simulink model "Scenario_MinimumExample_TwithoutTrafficLights"  (R2021a)
settings: Solver=VariableStepAuto  StartTime=0.0  StopTime=15  RelTol=1e-3
model workspace (MAT data in the model file):
  Kz_dif : Simulink.Parameter (value not decoded)
  Kz_il : Simulink.Parameter (value not decoded)
  Kz_ir : Simulink.Parameter (value not decoded)
  Kz_is : Simulink.Parameter (value not decoded)
  Kz_long : Simulink.Parameter (value not decoded)
  Kz_pre : Simulink.Parameter (value not decoded)
  L_dif : Simulink.Parameter (value not decoded)
  L_il : Simulink.Parameter (value not decoded)
  L_ir : Simulink.Parameter (value not decoded)
  L_is : Simulink.Parameter (value not decoded)
  L_long : Simulink.Parameter (value not decoded)
  L_pre : Simulink.Parameter (value not decoded)
  Lc : Simulink.Parameter (value not decoded)
  Rk : Simulink.Parameter (value not decoded)
  Tz_dif : Simulink.Parameter (value not decoded)
  Tz_il : Simulink.Parameter (value not decoded)
  Tz_ir : Simulink.Parameter (value not decoded)
  Tz_is : Simulink.Parameter (value not decoded)
  Tz_long : Simulink.Parameter (value not decoded)
  Tz_pre : Simulink.Parameter (value not decoded)
  ds : Simulink.Parameter (value not decoded)
  dt : Simulink.Parameter (value not decoded)
  v : Simulink.Parameter (value not decoded)
symbols that are objects in the model workspace (value not decoded): Kz_dif, Kz_il, Kz_ir, Kz_is, Kz_long, Kz_pre, Rk, Tz_dif, Tz_il, Tz_ir, Tz_is, Tz_long, Tz_pre
libraries: StreetLanesLibrary x72, EdgesLibrary x64, SourcesAndSinksLibrary x12
(part 2 of 3)

== stateflow chart Scenario_MinimumExample_TwithoutTrafficLights/Chart1 ==
  note: Notizen (mal auf Deutsch):
      | wenn an einer kante etwas anliegt und keine der stärkeren kanten etwas anliegen hat,
      | und die konfliktbereiche frei sind: schalte kante frei
      | <Ali 3> wird dominiert von <Cl 7> und <Cs 8> [Kreuzungen: <Brs Co> <Cl Ao> <Cs Bo>
      | <Ari 4> wird nicht dominiert [Kreuzungen: <Brs Co>
      | <Cl 7> wird dominiert von <Brs 11> und <Brs 12> [Kreuzungen: <Brs Co> <Brs Ao><Ali Bo>
      | <Cs 8> wird nicht dominiert [Kreuzungen: <Ali Bo>
      | <Brs 11> wird dominiert von <Ali 3> und <Ari 4> [Kreuzungen: <Brs Ao> <Ali Bo> <Ari Co>*<Cl Ao>
      | <Brs 12> wird nicht dominiert [Kreuzungen: <Cl Ao>
      |
      | Anmerkung: die einflüsse Brs11 und Brs12 behindern sich nicht. da beide kanten an
      | EIN UND DEMSELBEN SEGMENT liegen, und unsere 0.5:0.5 gewichtung schon suggeriert,
      | dass sich hier die autos "spalten", können sich die autos beim "Parallelen" fließen
      | in die segmente <Brs Co> und <Brs Ao> nicht wirklich in die quere kommen. Oder selbst wenn sie es
      | tun, können wir nichts dagegen unternehmen - wenn wir einem der pfade gegenüber dem anderen
      | priorität geben, wird bei dem anderen jeweils NIE etwas fließen. Damit müssen wir wohl leben :(
      |
      | a)
      | if [Ali > 0 && Cl == 0 && Cs == 0 && Brs_Co == 0 && Cl_Ao == 0 && Cs_Bo == 0]{enableAli3=1;}
      | else {enableAli3=0;}
      | b)
      | if [Ari > 0 && Brs_Co == 0]{enableAri4=1;}
      | else {enableAri4=0;}
      | c)
      | if [Cl > 0 && Brs == 0 && Brs_Co == 0 && Brs_Ao == 0 && Ali_Bo == 0]{enableCl7=1;}
      | else {enableCl7=0;}
      | d)
      | if [Cs > 0 && Ali_Bo == 0]{enableCs8=1;}
      | else {enableCs8=0;}
      | e)
      | if [Brs > 0 && Ali == 0 && Ari == 0 && Ali_Bo == 0 && Ari_Co == 0 && Cl_Ao]{enableBrs11=1;}
      | else {enableBrs11=0;}
      | f)
      | if [Brs > 0 && Cl_Ao == 0]{enableBrs12=1;}
      | else {enableBrs12=0;}
      |
      | Anmerkung: Da es im Falle [Ali > 0 && Brs > 0 && Cl > 0] einen deadlock gibt, müssen wir uns entscheiden, wer fahren darf.
      |
      | // Brs11 soll das fahrtrecht bekommen, um den fluss entlang der geraden aufrechtzuerhalten, wenn möglich
      | if [Ari == 0 && (Ali_Bo == 0 && Ari_Co == 0 && Cl_Ao == 0)]{enableBrs11=1;}
      | else
      |
      | // falls Brs12 nicht kann, versucht Ali zu fahren. Eigentlich müsste Cl die nächstbeste Wahl sein,
      | // allerdings kann Cl im falle eines Deadlocks ohnehin nicht fließen, da wegen unserer modellierung
      | // der 1x2 kanten (bzw. 1x2 segmente) gilt "Deadlock => [Brs > 0] => [Brs12 will aktiv sein]" - und da
      | // Brs12 vorrang vor Cl7 hat, ist Cl7 in diesem szenario grundsätzlich blockiert.
      | if [Cs == 0 && (Brs_Co == 0 && Cl_Ao == 0 && Cs_Bo == 0)]{enableAli3=1;}
      | else //guess noone can make it
  note: ?
  state InitiatePerStepCheck
  note: Brs-11-<Brs Co>-6-Co
      | (Links will geradeaus)
  note: Brs-12-<Brs Ao>-1-Ao
      | (Links will geradeaus)
  note: Ari-4-<Ari Co>-5-Co
      | (Unten will rechts abbiegen)
  note: Cl-7-<Cl Ao>-2-Ao
      | (Rechts will links abbiegen)
  note: Cs-8-<Cl Ao>-9-Bo
      | (Rechts will geradeaus)
  note: Ali-3-<Ali Bo>-10-Bo
      | (Unten will Links abbiegen)
  note: Deadlock-Detection
  note: Anstelle der ebene für deadlock resolution konnte man den "Links will geradeaus" bereich in der reihenfolge VOR "Unten will links abbiegen" setzen. "Links will geradeaus" muss dann um eine weitere kante mit höchster priorität ergänzt werden mit einem label
      | [ (Ali > 0 && Brs > 0 && Cl > 0 ) && (Ari == 0 && Ali_Bo == 0 && Ari_Co == 0]{enableBrs11=1;}
      |
      | "Unten will links abbiegen" wird dann ebenfalls um eine Kante mit höchster priorität ergänzt mit dem Label
      | [ (Ali > 0 && Brs > 0 && Cl > 0) && (Cs_Bo == 0 && Cl_Ao == 0) && ~(enableBrs11==1)
  note: Deadlock-Resolution
  InitiatePerStepCheck -> (junction 23) [order 1] : [Ali > 0 && Cl == 0 && Cs == 0 && Brs_Co == 0 && Cl_Ao == 0 && Cs_Bo == 0]
      | {enableAli3=1; }
  (junction 23) -> (junction 29) [order 1] : [Ari > 0 && Brs_Co == 0]{enableAri4=1;}
  (junction 29) -> (junction 36) [order 1] : [Cl > 0 && Brs == 0 && Brs_Co == 0 && Brs_Ao == 0 && Ali_Bo == 0]{enableCl7=1; }
  (junction 39) -> (junction 40) [order 1] : [Brs > 0 && Ali == 0 && Ari == 0 && Ali_Bo == 0 && Ari_Co == 0 && Cl_Ao]{enableBrs11=1;}
  (junction 40) -> (junction 45) [order 1] : [Brs > 0 && Cl_Ao == 0]{enableBrs12=1;}
  (junction 36) -> (junction 39) [order 1] : [Cs > 0 && Ali_Bo == 0]{enableCs8=1;}
  (junction 39) -> (junction 40) [order 2] : {enableBrs11=0;}
  (junction 29) -> (junction 36) [order 2] : {enableCl7=0;}
  (junction 36) -> (junction 39) [order 2] : {enableCs8=0;}
  (junction 23) -> (junction 29) [order 2] : {enableAri4=0;}
  (junction 40) -> (junction 45) [order 2] : {enableBrs12=0;}
  InitiatePerStepCheck -> (junction 23) [order 2] : {enableAli3=0;}
  (junction 45) -> (junction 53)
  (junction 53) -> InitiatePerStepCheck [order 2]
  (default) -> InitiatePerStepCheck : {enableAli3 = 0; enableAri4 = 0;
      | enableCl7 = 0; enableCs8 = 0;
      | enableBrs11 = 0; enableBrs12 = 0;}
  (junction 53) -> (junction 64) [order 1] : [Ali > 0 && Brs > 0 && Cl > 0]
  (junction 64) -> (junction 71) [order 1] : [Ari == 0 && (Ali_Bo == 0 && Ari_Co == 0 && Cl_Ao == 0)]{enableBrs11=1;}
  (junction 64) -> (junction 71) [order 2] : [Ari > 0 && Cs == 0 && (Brs_Co == 0 && Cl_Ao == 0 && Cs_Bo == 0)]{enableAli3=1;}
  (junction 71) -> InitiatePerStepCheck
  data: Ali input; Ari input; Cl input; Cs input; Brs input; Ali_Bo input; Ari_Co input; Cl_Ao input; Cs_Bo input; Brs_Co input; Brs_Ao input; enableAli3 output; enableAri4 output; enableCl7 output; enableCs8 output; enableBrs11 output; enableBrs12 output

== stateflow chart Scenario_MinimumExample_TwithoutTrafficLights/Plus-Controller ==
  note: ?
  state Group__Crs_Brs
  state Group__Cl_Bl
  state Group__Ars_Drs
  state Group__Al_Dl
  note: check
      | Crs straight
      | crossings
  note: check
      | Cl
      | crossings
  note: check
      | Ars straight
      | crossings
  note: check
      | Al
      | crossings
  note: check
      | Crs right
      | crossings
  note: check
      | Bl
      | crossings
  note: check
      | Ars right
      | crossings
  note: check
      | Dl
      | crossings
  note: check
      | Brs straight
      | crossings
  note: check
      | Drs straight
      | crossings
  note: check
      | Brs right
      | crossings
  note: check
      | Drs right
      | crossings
  Group__Al_Dl -> Group__Crs_Brs [order 2] : [[[after(green_duration_l, sec)]]]
      | {enAl = 0; enDl = 0;}
  Group__Ars_Drs -> Group__Al_Dl [order 1] : [[after(green_duration_sr, sec)]]
      | {enAs = 0; enAr = 0; enDs = 0; enDr = 0;}
  Group__Cl_Bl -> Group__Ars_Drs [order 1] : [after(green_duration_l, sec)]
      | {enCl = 0; enBl = 0;}
  Group__Crs_Brs -> Group__Cl_Bl [order 1] : [after(green_duration_sr, sec)]
      | {enCs = 0; enCr = 0; ...
      | enBs = 0; enBr = 0;}
  (default) -> Group__Crs_Brs : {enAl = 0; enAs = 0; enAr = 0;
      | enBl = 0; enBs = 0; enBr = 0;
      | enCl = 0; enCs = 0; enCr = 0;
      | enDl = 0; enDs = 0; enDr = 0;}
  Group__Crs_Brs -> (junction 51) [order 2]
  (junction 109) -> Group__Crs_Brs
  Group__Cl_Bl -> (junction 117) [order 2]
  (junction 126) -> Group__Cl_Bl
  Group__Ars_Drs -> (junction 134) [order 2]
  (junction 131) -> Group__Ars_Drs
  Group__Al_Dl -> (junction 151) [order 1]
  (junction 160) -> Group__Al_Dl
  (junction 117) -> (junction 116) [order 2] : {enCl = 0;}
  (junction 51) -> (junction 59) [order 1] : [(Dl_Co==0 && Drs_Ao==0 ...
      | && Drs_Bo==0 && Bl_Do==0 ...
      | && Al_Bo==0 && Ars_Do==0)]
      | {enCs = 1;}
  (junction 117) -> (junction 116) [order 1] : [(Dl_Co==0 && Drs_Ao==0 && ....
      | Brs_Co==0 && Al_Bo==0 && ...
      | Ars_Do==0)]{enCl = 1;}
  (junction 51) -> (junction 59) [order 2] : {enCs = 0;}
  (junction 134) -> (junction 133) [order 1] : [((Cl_Ao==0 && Crs_Bo==0 && ...
      | Crs_Do==0 && Dl_Co==0 && ...
      | Bl_Do==0 && Brs_Co==0))]
      | {enAs = 1;}
  (junction 151) -> (junction 150) [order 1] : [(Cl_Ao==0 && Crs_Bo==0 ...
      | && Drs_Ao==0 && Bl_Do==0 ...
      | && Brs_Co==0)]{enAl = 1;}
  (junction 134) -> (junction 133) [order 2] : {enAs = 0;}
  (junction 151) -> (junction 150) [order 2] : {enAl = 0;}
  (junction 59) -> (junction 104) [order 1] : [(Ars_Do==0 && Bl_Do==0)]
      | {enCr = 1;}
  (junction 116) -> (junction 126) [order 1] : [(Al_Bo==0 && Ars_Do==0 && ...
      | Crs_Bo==0 && Dl_Co==0 && ...
      | Drs_Ao==0)]{enBl = 1;}
  (junction 59) -> (junction 104) [order 2] : {enCr = 0;}
  (junction 116) -> (junction 126) [order 2] : {enBl = 0;}
  (junction 133) -> (junction 143) [order 1] : [(Brs_Co==0 && Dl_Co==0)]
      | {enAr = 1;}
  (junction 150) -> (junction 160) [order 1] : [(Bl_Do==0 && Brs_Co==0 ...
      | && Ars_Do==0 && Cl_Ao==0 ...
      | && Crs_Bo==0)]{enDl = 1;}
  (junction 133) -> (junction 143) [order 2] : {enAr = 0;}
  (junction 150) -> (junction 160) [order 2] : {enDl = 0;}
  (junction 104) -> (junction 105) [order 1] : [(Al_Bo==0 && Ars_Do==0 ...
      | && Ars_Co==0 && Cl_Ao==0 ...
      | && Dl_Co==0 && Drs_Ao==0)]
      | {enBs = 1;}
  (junction 104) -> (junction 105) [order 2] : {enBs = 0;}
  (junction 143) -> (junction 141) [order 1] : [(Bl_Do==0 && Brs_Co==0 ...
      | && Brs_Ao==0 && Al_Bo==0 ...
      | && Cl_Ao==0 && Crs_Bo==0)]
      | {enDs = 1;}
  (junction 143) -> (junction 141) [order 2] : {enDs=0;}
  (junction 105) -> (junction 109) [order 1] : [Drs_Ao==0 && Cl_Ao==0]
      | {enBr = 1;}
  (junction 105) -> (junction 109) [order 2] : {enBr = 0;}
  (junction 141) -> (junction 131) [order 1] : [(Crs_Bo==0 && Al_Bo==0)]
      | {enDr = 1;}
  (junction 141) -> (junction 131) [order 2] : {enDr = 0;}
  data: Bl input; Brs input; Al input; Ars input; Cl input; Crs input; Dl input; Drs input; Al_Bo input; Ars_Do input; Ars_Co input; Bl_Do input; Brs_Co input; Brs_Ao input; Cl_Ao input; Crs_Bo input; Crs_Do input; Dl_Co input; Drs_Ao input; Drs_Bo input; enAl output =0; enAs output =0; enAr output =0; enBl output =0; enBs output =0; enBr output =0; enCl output =0; enCs output =0; enCr output =0; enDl output =0; enDs output =0; enDr output =0; green_duration_sr parameter; green_duration_l parameter
